simulink library "StateMachine"  (R2024a)
settings: Solver=VariableStepAuto  StartTime=0.0  StopTime=10.0  RelTol=1e-3
values from neighbouring files (symbols this model uses):
  VehicleState : value not decoded    [StateMachine.sldd]
undefined symbols (not defined in the file or in its folder): dt
libraries: simulink x2, Utilities x1
settings Model: RaptorUIDSize=4  Creator=serga  LastModifiedBy=serga

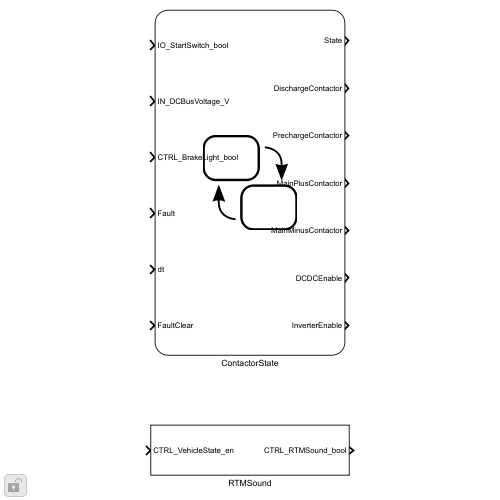
[thumbnail: Simulink's stored preview of the top-level diagram]
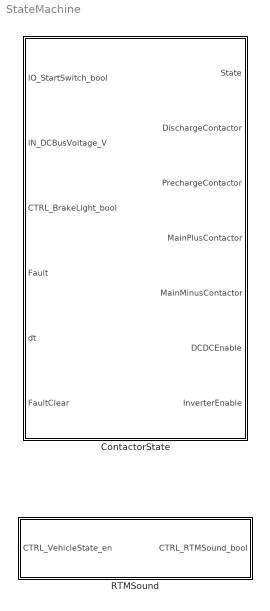
== system StateMachine ==
  ContactorState : Stateflow chart  TreatAsAtomicUnit=on
  RTMSound : Subsystem

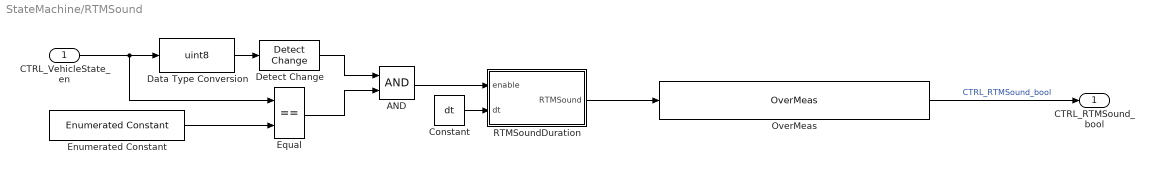
== system StateMachine/RTMSound ==
  CTRL_VehicleState_en : Inport
  AND : Logic  AllPortsSameDT=off  OutDataTypeStr=boolean
  Constant : Constant  Value=dt
  Data Type Conversion : DataTypeConversion  OutDataTypeStr=uint8  SaturateOnIntegerOverflow=off  RndMeth=Floor
  Detect Change : simulink/Logic and Bit Operations/Detect Change  vinit=0  OutDataTypeStr=boolean
  Enumerated Constant : simulink/Sources/Enumerated Constant  OutDataTypeStr=Enum: VehicleState  Value=VehicleState.ReadyToMove  SampleTime=inf
  Equal : RelationalOperator  Operator===  OutDataTypeStr=boolean  RndMeth=Simplest  InputSameDT=off
  OverMeas : Utilities/OverMeas  sigName='CTRL_RTMSound_bool'  minimum=0  maximum=1
  RTMSoundDuration : Stateflow chart  TreatAsAtomicUnit=on
  CTRL_RTMSound_bool : Outport
  wires:
  OverMeas/1 -> CTRL_RTMSound_bool/1  "CTRL_RTMSound_bool"
  Detect Change/1 -> AND/1
  Enumerated Constant/1 -> Equal/2
  CTRL_VehicleState_en/1 -> Data Type Conversion/1, Equal/1
  Data Type Conversion/1 -> Detect Change/1
  Equal/1 -> AND/2
  AND/1 -> RTMSoundDuration/1(enable)
  Constant/1 -> RTMSoundDuration/2(dt)
  RTMSoundDuration/1(RTMSound) -> OverMeas/1

== stateflow chart StateMachine/RTMSound/RTMSoundDuration ==
  state RTMSoundStop
    en:
    RTMSound = false;
    timer = 0;
  state RTMSoundStart
    en:
    RTMSound = true;
    du:
    timer = timer + dt;
  (default) -> RTMSoundStop
  RTMSoundStop -> RTMSoundStart : [enable == true]
  RTMSoundStart -> RTMSoundStop : [timer > 200]
  data: RTMSound output =false; enable input; timer local single; dt input

== stateflow chart StateMachine/ContactorState ==
  state Normal
    state Precharge
      state StartDelay
        en:
        timer = 0;
        State = VehicleState.StartDelay;
        du:
        timer = timer + dt;
      note: if there is already accumulator voltage present before even actuating the contactors, then a contactor has been welded
      note: about 1 sec to discharge to 60V
      state PrechargeReady
        % waiting for tractive system switch signal
        en:
        State = VehicleState.PrechargeReady;
        MainPlusContactor = ContactorState.Open;
        MainMinusContactor = ContactorState.Open;
        PrechargeContactor = ContactorState.Open;
        DischargeContactor = ContactorState.Close;
        DCDCEnable = DCDCStatus.Off;
        InverterEnable = InverterStatus.Off;
        timer = 0;
      state PrechargeTimeout
        % timed out, retry
        en:
        State = VehicleState.PrechargeTimeout
        MainPlusContactor = ContactorState.Open;
        MainMinusContactor = ContactorState.Open;
        PrechargeContactor = ContactorState.Open;
        DischargeContactor = ContactorState.Close;
        DCDCEnable = DCDCStatus.Off;
        InverterEnable = InverterStatus.Off;
        timer = 0;
        du:
        timer = timer + dt;
      state PrechargeBegin
        en:
        State = VehicleState.Precharge;
        DischargeContactor = ContactorState.Open;
        PrechargeContactor = ContactorState.Close;
        MainMinusContactor = ContactorState.Close;
        timer = 0;
      state PrechargeWait
        % after closing the contactor, start the precharge timer
        du:
        timer = timer + dt;
      note: change to something else -- this is just for testing
      state PrechargeComplete
        en:
        State = VehicleState.PrechargeComplete;
        timer = 0;
      (default) -> StartDelay
      StartDelay -> PrechargeReady : [timer >  500 ...
          | && Fault == false]
      (junction 38) -> PrechargeReady
      PrechargeTimeout -> (junction 38) : [timer >  500]
      PrechargeReady -> PrechargeBegin [order 2]
      PrechargeBegin -> PrechargeWait
      (junction 27) -> PrechargeTimeout
      PrechargeWait -> (junction 27) [order 2] : [timer >  15000]
      PrechargeWait -> PrechargeComplete [order 1] : [IN_DCBusVoltage_V > 260]
    state ReadyToMove
      state RTM
        en:
        State = VehicleState.ReadyToMove;
        MainPlusContactor = ContactorState.Close;
        PrechargeContactor = ContactorState.Open;
        InverterEnable = InverterStatus.On;
        DCDCEnable = DCDCStatus.On;
        timer = 0;
      state Standby
        % wait for all conditions to be satisfied
        en:
        State = VehicleState.Standby;
        du:
        timer = timer + dt;
      (default) -> Standby
      Standby -> RTM : [DischargeContactor == ContactorState.Open ...
          | && PrechargeContactor == ContactorState.Close ...
          | && MainMinusContactor == ContactorState.Close ...
          | && CTRL_BrakeLight_bool == true ...
          | && IO_StartSwitch_bool == true]
    (default) -> Precharge
    PrechargeComplete -> ReadyToMove : [DischargeContactor == ContactorState.Open ...
        | && MainMinusContactor == ContactorState.Close]
  note: watch for voltage sag
  state Faulted
    en:
    State = VehicleState.Faulted;
    MainPlusContactor = ContactorState.Open;
    MainMinusContactor = ContactorState.Open;
    PrechargeContactor = ContactorState.Open;
    DischargeContactor = ContactorState.Close;
    DCDCEnable = DCDCStatus.Off;
    InverterEnable = InverterStatus.Off;
    timer = 0;
  (default) -> Normal
  (junction 119) -> Normal
  Faulted -> (junction 119)
  PrechargeReady -> (junction 104) [order 1] : [duration(IN_DCBusVoltage_V > 60) > 2]
  (junction 104) -> Faulted
  ReadyToMove -> Faulted : [IN_DCBusVoltage_V < 230 ...
      | || IN_DCBusVoltage_V > 405]
  Normal -> Faulted : [Fault == true]
  data: State output; IO_StartSwitch_bool input; DischargeContactor output; PrechargeContactor output; MainPlusContactor output; MainMinusContactor output; timer local single; IN_DCBusVoltage_V input; CTRL_BrakeLight_bool input; Fault input; dt input; DCDCEnable output; InverterEnable output; FaultClear input
